simulink model "illMatrixModel"  (R2022a)
settings: Solver=ode113  StartTime=0.0  StopTime=1.3  MaxStep=1e-3  RelTol=1e-3
libraries: simulink x1
settings Model: Creator=Administrator  LastModifiedBy=Administrator

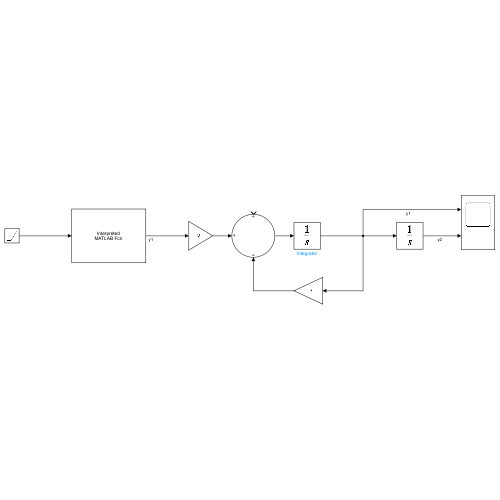
[thumbnail: Simulink's stored preview of the top-level diagram]
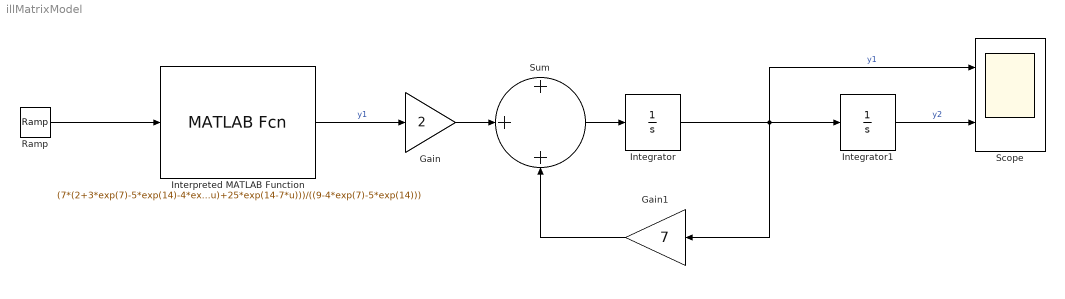
== system illMatrixModel ==
  Gain : Gain  Gain=2
  Gain1 : Gain  Gain=7
  Integrator : Integrator  InitialCondition=3
  Integrator1 : Integrator  InitialCondition=1
  Interpreted MATLAB Function : MATLABFcn  MATLABFcn=(7*(2+3*exp(7)-5*exp(14)-4*exp(7-7*u)+25*exp(14-7*u)))/((9-4*exp(7)-5*exp(14)))  OutputDimensions=1
  Ramp : simulink/Sources/Ramp  slope=1  start=0  InitialOutput=0
  Scope : Scope  NumInputPorts=2
  Sum : Sum  Inputs=+++
  wires:
  Ramp/1 -> Interpreted MATLAB Function/1
  Interpreted MATLAB Function/1 -> Gain/1  "y1"
  Sum/1 -> Integrator/1
  Gain/1 -> Sum/2
  Integrator/1 -> Scope/1, Integrator1/1, Gain1/1  "y1"
  Gain1/1 -> Sum/3
  Integrator1/1 -> Scope/2  "y2"
